simulink model "Test_Step_Ramp"  (R2024a)
settings: Solver=VariableStepAuto  StartTime=0.0  StopTime=10.0  RelTol=1e-3
undefined symbols (not defined in the file): Gain_Derivative_Controller, Gain_Integral_Controller, Gain_Proportional_Controller
libraries: simulink x1, cstblocks x1
settings Model: Creator=gerar  LastModifiedBy=gerar

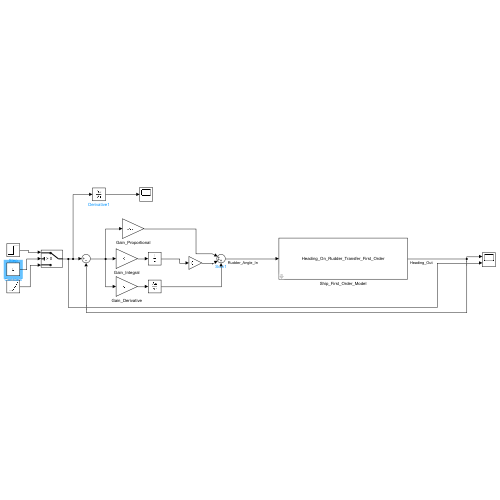
[thumbnail: Simulink's stored preview of the top-level diagram]
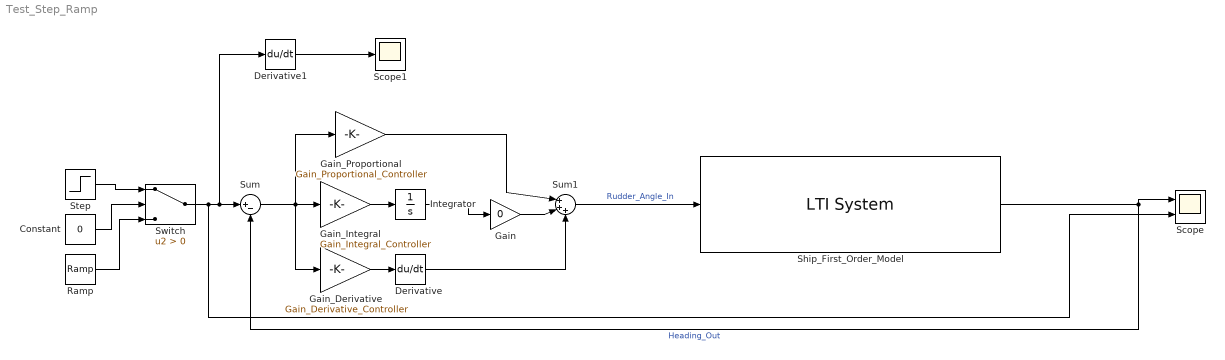
== system Test_Step_Ramp ==
  Constant : Constant  Value=0
  Derivative : Derivative
  Derivative1 : Derivative
  Gain : Gain  Gain=0
  Gain_Derivative : Gain  Gain=Gain_Derivative_Controller
  Gain_Integral : Gain  Gain=Gain_Integral_Controller
  Gain_Proportional : Gain  Gain=Gain_Proportional_Controller
  Integrator : Integrator
  Ramp : simulink/Sources/Ramp  slope=5*(pi/180)  start=1  InitialOutput=0
  Scope : Scope  NumInputPorts=2
  Scope1 : Scope
  Ship_First_Order_Model : cstblocks/LTI System  sys=Heading_On_Rudder_Transfer_First_Order  IC=[]  PadeOrder=0
  Step : Step  After=5*(pi/180)  SampleTime=0
  Sum : Sum  Inputs=|+-
  Sum1 : Sum  Inputs=|+++
  Switch : Switch  Criteria=u2 > Threshold  SaturateOnIntegerOverflow=off  InputSameDT=off
  wires:
  Sum/1 -> Gain_Proportional/1, Gain_Derivative/1, Gain_Integral/1
  Sum1/1 -> Ship_First_Order_Model/1  "Rudder_Angle_In"
  Gain_Integral/1 -> Integrator/1
  Derivative/1 -> Sum1/3
  Gain_Derivative/1 -> Derivative/1
  Gain_Proportional/1 -> Sum1/1
  Integrator/1 -> Gain/1
  Ship_First_Order_Model/1 -> Scope/1, Sum/2  "Heading_Out"
  Gain/1 -> Sum1/2
  Switch/1 -> Scope/2, Derivative1/1, Sum/1
  Step/1 -> Switch/1
  Constant/1 -> Switch/2
  Ramp/1 -> Switch/3
  Derivative1/1 -> Scope1/1
